simulink model "NEWVSG"  (R2024b)
settings: Solver=FixedStepAuto  StartTime=0.0  StopTime=2  FixedStep=1e-6  RelTol=1e-3
InitFcn:
  | fn=50;
  | Un=24;
  | Sb=100;
  | Qref=1;
  | w0=2*pi*fn;
  | Pref=100;
  | J=0.0002;%典型值0.00002
  | D=0.4;%典型值0.4
  | kp=0.5;%典型值1
  | kv=0.24;%典型值1 对无功调节响应变快，振荡增加
  | kq=0.01;%典型值0.01 增大此值对无功响应没有影响，随意增大会试系统振荡
libraries: spsSeriesRLCBranchLib x6, spsVoltageMeasurementLib x4, slpidlib x2, spsACVoltageSourceLib x1, spsBreakerLib x1, spspowerguiLib x1, spsCurrentMeasurementLib x1, spsDCVoltageSourceLib x1, powerlib_extras x1, simulink x1, spsUniversalBridgeLib x1, spsRMSLib x1
settings Model: Creator=ASUS  LastModifiedBy=ASUS
settings DataIOCC: ReturnWorkspaceOutputs=off

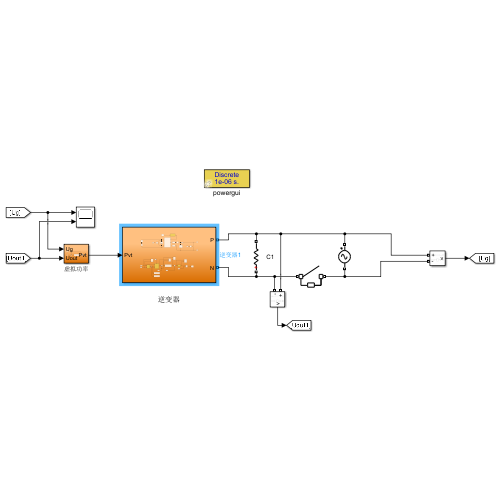
[thumbnail: Simulink's stored preview of the top-level diagram]
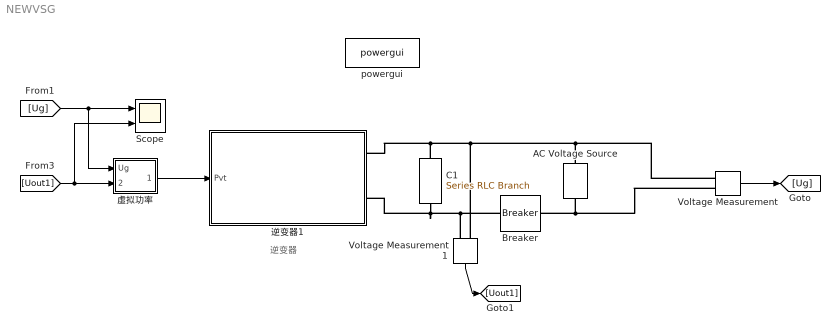
== system NEWVSG ==
  note: 逆变器
  AC Voltage Source : spsACVoltageSourceLib/AC Voltage Source  Amplitude=24*sqrt(2)  Phase=180  Frequency=50  SampleTime=0  Measurements=None  BusType=swing  Pref=10e3  Qref=0  Qmin=-inf  Qmax=+inf
  Breaker : spsBreakerLib/Breaker  InitialState=0  SwitchingTimes=[0.5 1.5 2]  External=off  BreakerResistance=0.01  SnubberResistance=1e6  SnubberCapacitance=inf  Measurements=None  MoreParameters=on  NoBreakLoop=off
  C1 : spsSeriesRLCBranchLib/Series RLC Branch  LConnTagsString=__new0  RConnTagsString=__new0  BranchType=R  Resistance=5  Inductance=0  SetiL0=off  InitialCurrent=0  Capacitance=3e-6  Setx0=off  InitialVoltage=350  Measurements=None
  Scope : Scope  NumInputPorts=2
  Voltage Measurement : spsVoltageMeasurementLib/Voltage Measurement  PhasorSimulation=off  OutputType=Complex  PSBequivalent=0
  Voltage Measurement1 : spsVoltageMeasurementLib/Voltage Measurement  PhasorSimulation=off  OutputType=Complex  PSBequivalent=0
  powergui : spspowerguiLib/powergui  SimulationMode=Discrete  SampleTime=1e-6  frequency=60  Iterations=50  frequencyindice=50  Pbase=100e6  ErrMax=1e-4  UnitsV=kV  UnitsW=MW  buscounter=0  FunctionMessages=off  echomessages=off  EnableUseOfTLC=off  CurrentSourceSwitches=off  DisableSnubberDevices=off  DisableRonSwitches=off  DisableVfSwitches=off  DisplayEquations=off  AutomaticDiscreteSolvers=off  SolverType=Tustin/Backward Euler (TBE)  Interpol=off  ExternalGateDelay=off  methode=off  Ts=0  x0status=blocks  SPID=off  SwTol=0  HookPort=off  NonlinearTolerance=1e-4  nMaxIteration=100  ContinueOnMaxIteration=off  RestoreLinks=warning  ResistiveCurrentMeasurement=off  Frange=[0:2:500]  Ylog=off  Xlog=on  ShowGrid=off  save=off  variable=ZData  structure=QQQQQ  ZoomFFT=off  StartTime=0.5  cycles=15  DisplayStyle=1  fundamental=50  FreqAxis=off  MaxFrequency=1000  frequencyindicesteady=1  RmsSteady=1  display=off
  虚拟功率 : Subsystem
  逆变器1 : Subsystem
      settings: PortSchema="{\"entries\":[{\"content\":{\"sides\":[{\"content\":{},\"type\":\"ConnectorPlacement.EquallySpacedRectSide\",\"uuid\":\"a93680c0-663f-4f34-b987-d4dbc78c4730\"},{\"content\":{\"side\":\"RIGHT\"},\"type\":\"ConnectorPlacement.EquallySpacedRectSide\",\"uuid\":\"c51b779d-273d-4c0b-b109-877d58986348\"},{\"content\":{\"connectorIds\":[\"In1\"],\"side\":\"TOP\"},\"type\":\"ConnectorPlacement.EquallySpacedRectSide\",\"uuid\":\"2562aadc-3010-41da-9435-a9c5d6d596bf\"},{\"content\":{\"connectorIds\":[\"RConn1\",\"RConn2\"],\"side\":\"BOTTOM\"},\"type\":\"ConnectorPlacement.EquallySpacedRectSide\",\"uuid\":\"37d810f6-ab81-4958-8785-8b1d526c8ea4\"}]},\"type\":\"ConnectorPlacement.EquallySpacedConnector\",\"uuid\":\"534c4e7c-1935-4667-a56d-b399c5878ac6\"}],\"packageUris\":[\"http://schema.mathworks.com/mf0/Connector/R2020b\"],\"version\":\"1.0\"}"
  wires:
  虚拟功率/1(Pvt) -> 逆变器1/1(Pvt)
  [Uout1] -> 虚拟功率/2(Uout), Scope/2
  [Ug] -> 虚拟功率/1(Ug), Scope/1
  Voltage Measurement1/1 -> [Uout1]
  Voltage Measurement/1 -> [Ug]
  connections:
  AC Voltage Source/LConn1 -- Breaker/RConn1 -- Voltage Measurement/LConn2
  AC Voltage Source/RConn1 -- 逆变器1/RConn2 -- C1/RConn1 -- Voltage Measurement1/LConn1 -- Voltage Measurement/LConn1
  Breaker/LConn1 -- 逆变器1/RConn1 -- C1/LConn1 -- Voltage Measurement1/LConn2

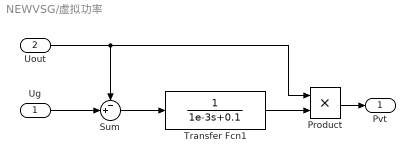
== system NEWVSG/虚拟功率 ==
  Ug : Inport
  Uout : Inport  Port=2
  Product : Product
  Sum : Sum  Inputs=-+|
  Transfer Fcn1 : TransferFcn  Denominator=[1e-3 0.1]
  Pvt : Outport
  wires:
  Transfer Fcn1/1 -> Product/2
  Uout/1 -> Sum/1, Product/1
  Ug/1 -> Sum/2
  Sum/1 -> Transfer Fcn1/1
  Product/1 -> Pvt/1

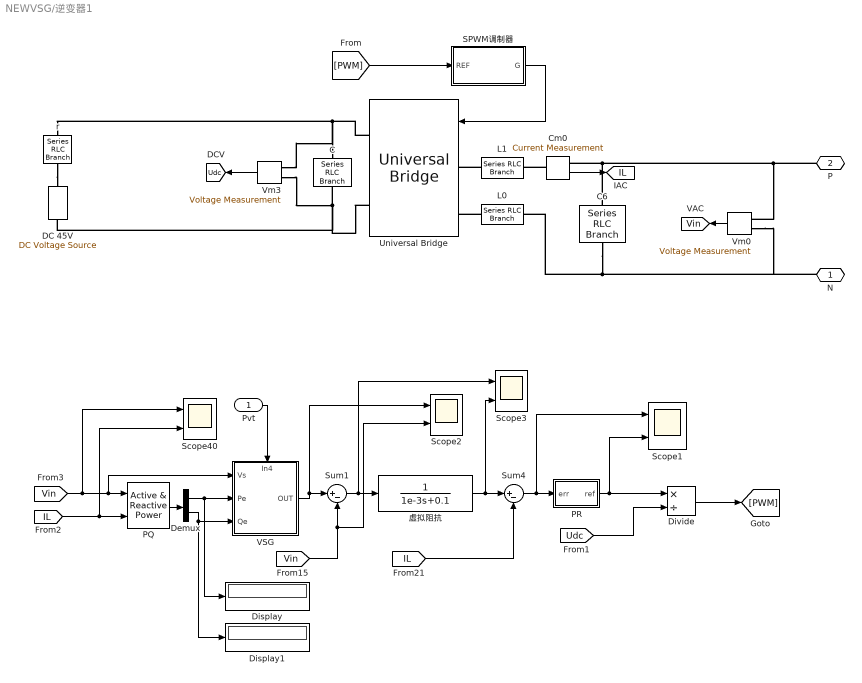
== system NEWVSG/逆变器1 ==
  Pvt : Inport
  C : spsSeriesRLCBranchLib/Series RLC Branch  LConnTagsString=__new0  RConnTagsString=__new0  BranchType=C  Resistance=0.05  Inductance=0  SetiL0=off  InitialCurrent=0  Capacitance=4e-3  Setx0=on  InitialVoltage=45  Measurements=None
  C6 : spsSeriesRLCBranchLib/Series RLC Branch  LConnTagsString=__new0  RConnTagsString=__new0  BranchType=RC  Resistance=1  Inductance=0  SetiL0=off  InitialCurrent=0  Capacitance=3e-6  Setx0=off  InitialVoltage=350  Measurements=None
  Cm0 : spsCurrentMeasurementLib/Current Measurement  PhasorSimulation=off  OutputType=Complex  PSBequivalent=0
  DC 45V : spsDCVoltageSourceLib/DC Voltage Source  Amplitude=45  Measurements=None
  Demux : Demux  Outputs=2
  Display : Display
  Display1 : Display
  Divide : Product  Inputs=*/
  L0 : spsSeriesRLCBranchLib/Series RLC Branch  LConnTagsString=__new0  RConnTagsString=__new0  BranchType=RL  Resistance=81e-3  Inductance=5e-4  SetiL0=off  InitialCurrent=0  Capacitance=inf  Setx0=off  InitialVoltage=0  Measurements=None
  L1 : spsSeriesRLCBranchLib/Series RLC Branch  LConnTagsString=__new0  RConnTagsString=__new0  BranchType=RL  Resistance=81e-3  Inductance=5e-4  SetiL0=off  InitialCurrent=0  Capacitance=inf  Setx0=off  InitialVoltage=0  Measurements=None
  PQ : powerlib_extras/Measurements/Active & Reactive Power  f1=50
  PR : Subsystem  TreatAsAtomicUnit=on  mask{Kp=4, Kr=100, Wc=20, Upper=10000, Lower=-10000}
  SPWM调制器 : Subsystem
  Scope{1..3,40} (4 alike) : Scope  NumInputPorts=2
  Sum1 : Sum  Inputs=|+-
  Sum4 : Sum  Inputs=|+-
  Universal Bridge : spsUniversalBridgeLib/Universal Bridge  Arms=2  SnubberResistance=1e5  SnubberCapacitance=inf  Device=MOSFET / Diodes  Ron=0.01  Lon=0  ForwardVoltages="[  0  0  ]"  ForwardVoltage=0  GTOparameters=[ 10e-6 , 20e-6 ]  IGBTparameters=[ 1e-6 , 2e-6 ]  Measurements=None  Measurements_2=None  converterType=Rectifier
  VSG : Subsystem
      settings: PortSchema="{\"entries\":[{\"content\":{\"sides\":[{\"content\":{\"connectorIds\":[\"In1\",\"In2\",\"In3\"]},\"type\":\"ConnectorPlacement.EquallySpacedRectSide\",\"uuid\":\"aa52da4d-f934-47f0-800a-70195eace23d\"},{\"content\":{\"connectorIds\":[\"Out1\"],\"side\":\"RIGHT\"},\"type\":\"ConnectorPlacement.EquallySpacedRectSide\",\"uuid\":\"90c9e631-faf7-42fe-9625-64aab78a5d50\"},{\"content\":{\"connectorIds\":[\"In4\"],\"side\":\"TOP\"},\"type\":\"ConnectorPlacement.EquallySpacedRectSide\",\"uuid\":\"027d9aee-22b5-4ed3-abeb-2e992649b09d\"}]},\"type\":\"ConnectorPlacement.EquallySpacedConnector\",\"uuid\":\"8c25c37b-9c43-4192-89c9-033fe8e08717\"}],\"packageUris\":[\"http://schema.mathworks.com/mf0/Connector/R2020b\"],\"version\":\"1.0\"}"
  Vm0 : spsVoltageMeasurementLib/Voltage Measurement  PhasorSimulation=off  OutputType=Complex  PSBequivalent=0
  Vm3 : spsVoltageMeasurementLib/Voltage Measurement  PhasorSimulation=off  OutputType=Complex  PSBequivalent=0
  r : spsSeriesRLCBranchLib/Series RLC Branch  LConnTagsString=__new0  RConnTagsString=__new0  BranchType=R  Resistance=0.05  Inductance=0  SetiL0=off  InitialCurrent=0  Capacitance=2e-3  Setx0=on  InitialVoltage=390  Measurements=None
  虚拟阻抗 : TransferFcn  Denominator=[1e-3 0.1]
  N : PMIOPort  Side=Right
  P : PMIOPort  Port=2  Side=Right
  tag scope: IL=global, Udc=global, Vin=global
  wires:
  Vm0/1 -> [Vin]
  Cm0/1 -> [IL]
  Vm3/1 -> [Udc]
  Sum4/1 -> PR/1(err), Scope1/1
  PR/1(ref) -> Divide/1, Scope1/2
  [Udc] -> Divide/2
  [IL] -> Sum4/2
  SPWM调制器/1(G) -> Universal Bridge/1
  [IL] -> PQ/2, Scope40/2
  PQ/1 -> Demux/1
  Sum1/1 -> Scope3/1, 虚拟阻抗/1
  [Vin] -> PQ/1, VSG/1(Vs), Scope40/1
  Demux/1 -> VSG/2(Pe), Display/1
  Demux/2 -> VSG/3(Qe), Display1/1
  [Vin] -> Sum1/2, Scope2/2
  Divide/1 -> [PWM]
  [PWM] -> SPWM调制器/1(REF)
  VSG/1(OUT) -> Scope2/1, Sum1/1
  Pvt/1 -> VSG/4(In4)
  虚拟阻抗/1 -> Scope3/2, Sum4/1
  connections:
  L0/LConn1 -- Universal Bridge/LConn2
  L1/LConn1 -- Universal Bridge/LConn1
  P/RConn1 -- Vm0/LConn1 -- Cm0/RConn1 -- C6/LConn1
  Cm0/LConn1 -- L1/RConn1
  C6/RConn1 -- Vm0/LConn2 -- N/RConn1 -- L0/RConn1
  r/RConn1 -- DC 45V/RConn1
  Vm3/LConn2 -- Universal Bridge/RConn2 -- DC 45V/LConn1 -- C/RConn1
  Universal Bridge/RConn1 -- Vm3/LConn1 -- C/LConn1 -- r/LConn1

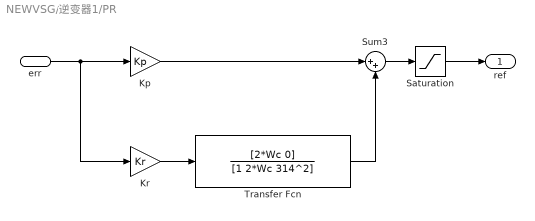
== system NEWVSG/逆变器1/PR ==
  err : Inport
  Kp : Gain  Gain=Kp
  Kr : Gain  Gain=Kr
  Saturation : Saturate  UpperLimit=Upper  LowerLimit=Lower
  Sum3 : Sum  Inputs=|++
  Transfer Fcn : TransferFcn  Numerator=[2*Wc 0]  Denominator=[1 2*Wc 314^2]
  ref : Outport
  wires:
  Kp/1 -> Sum3/1
  Sum3/1 -> Saturation/1
  err/1 -> Kr/1, Kp/1
  Kr/1 -> Transfer Fcn/1
  Transfer Fcn/1 -> Sum3/2
  Saturation/1 -> ref/1

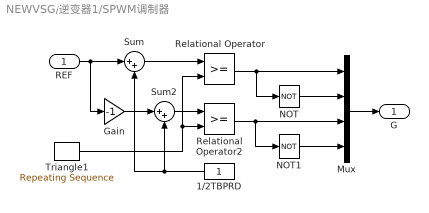
== system NEWVSG/逆变器1/SPWM调制器 ==
  REF : Inport
  1/2TBPRD : Constant
  Gain : Gain  Gain=-1
  Mux : Mux
  NOT : Logic  Operator=NOT  IconShape=distinctive  AllPortsSameDT=off  OutDataTypeStr=boolean
  NOT1 : Logic  Operator=NOT  IconShape=distinctive  AllPortsSameDT=off  OutDataTypeStr=boolean
  Relational Operator : RelationalOperator  OutDataTypeStr=boolean  InputSameDT=off
  Relational Operator2 : RelationalOperator  OutDataTypeStr=boolean  InputSameDT=off
  Sum : Sum  Inputs=|++
  Sum2 : Sum  Inputs=|++
  Triangle1 : simulink/Sources/Repeating Sequence  rep_seq_t=[0 1/16000/2 1/16000]  rep_seq_y=[0 2 0]
  G : Outport
  wires:
  Triangle1/1 -> Relational Operator2/2, Relational Operator/2
  Sum/1 -> Relational Operator/1
  REF/1 -> Gain/1, Sum/1
  Gain/1 -> Sum2/1
  Sum2/1 -> Relational Operator2/1
  1/2TBPRD/1 -> Sum/2, Sum2/2
  Relational Operator/1 -> NOT/1, Mux/1
  NOT/1 -> Mux/2
  Mux/1 -> G/1
  NOT1/1 -> Mux/4
  Relational Operator2/1 -> NOT1/1, Mux/3

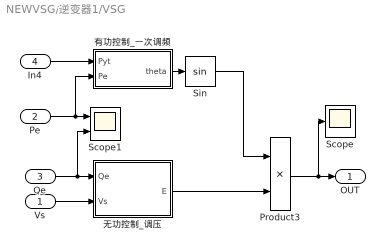
== system NEWVSG/逆变器1/VSG ==
  Vs : Inport
  Pe : Inport  Port=2
  Qe : Inport  Port=3
  In4 : Inport  Port=4
  Product3 : Product
  Scope : Scope
  Scope1 : Scope  NumInputPorts=2
  Sin : Trigonometry
  无功控制_调压 : Subsystem
  有功控制_一次调频 : Subsystem
  OUT : Outport
  wires:
  Pe/1 -> 有功控制_一次调频/2(Pe), Scope1/1
  Product3/1 -> Scope/1, OUT/1
  无功控制_调压/1(E) -> Product3/2
  有功控制_一次调频/1(theta) -> Sin/1
  Sin/1 -> Product3/1
  Qe/1 -> Scope1/2, 无功控制_调压/1(Qe)
  Vs/1 -> 无功控制_调压/2(Vs)
  In4/1 -> 有功控制_一次调频/1(Pyt)

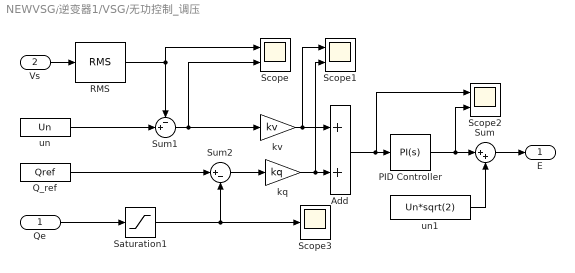
== system NEWVSG/逆变器1/VSG/无功控制_调压 ==
  Qe : Inport
  Vs : Inport  Port=2
  Add : Sum
  PID Controller : slpidlib/PID Controller  Controller=PI  Form=Parallel  TimeDomain=Continuous-time  UseExternalTs=off  SampleTime=-1  IntegratorMethod=Forward Euler  FilterMethod=Forward Euler  ControllerParametersSource=internal  P=0.1  I=50  UseKiTs=off  D=0  UseExternalDerivativeSource=off  N=100  UseFilter=on  TunerSelectOption=Transfer Function Based (PID Tuner App)  InitialConditionSource=internal  InitialConditionForIntegrator=0  InitialConditionForFilter=0  DifferentiatorICPrevScaledInput=0  ExternalReset=none  TrackingMode=off  Kt=1  LimitOutput=off  SatLimitsSource=internal  UpperSaturationLimit=inf  LowerSaturationLimit=-inf  LinearizeAsGain=on  AntiWindupMode=none  Kb=1  LimitIntegrator=off  UpperIntegratorSaturationLimit=inf  LowerIntegratorSaturationLimit=-inf  POutMin=[]  POutMax=[]  IOutMin=[]  IOutMax=[]  DOutMin=[]  DOutMax=[]  NOutMin=[]  NOutMax=[]  SumOutMin=[]  SumOutMax=[]  SaturationOutMin=[]  SaturationOutMax=[]  PParamMin=[]  PParamMax=[]  IParamMin=[]  IParamMax=[]  DParamMin=[]  DParamMax=[]  NParamMin=[]  NParamMax=[]  KbParamMin=[]  KbParamMax=[]  KtParamMin=[]  KtParamMax=[]  KbOutMin=[]  KbOutMax=[]  KtOutMin=[]  KtOutMax=[]  IntegratorOutMin=[]  IntegratorOutMax=[]  FilterOutMin=[]  FilterOutMax=[]  SumI1OutMin=[]  SumI1OutMax=[]  SumI2OutMin=[]  SumI2OutMax=[]  SumI3OutMin=[]  SumI3OutMax=[]  SumI4OutMin=[]  SumI4OutMax=[]  SumDOutMin=[]  SumDOutMax=[]  DifferentiatorOutMin=[]  DifferentiatorOutMax=[]  FilterDiffOutCoefMin=[]  FilterDiffOutCoefMax=[]  ReciprocalOutMin=[]  ReciprocalOutMax=[]  SumDenOutMin=[]  SumDenOutMax=[]  SumNumOutMin=[]  SumNumOutMax=[]  DivideOutMin=[]  DivideOutMax=[]  UdiffTsProdOutMin=[]  UdiffTsProdOutMax=[]  NTsProdOutMin=[]  NTsProdOutMax=[]  UintegralTsProdOutMin=[]  UintegralTsProdOutMax=[]  UngainTsProdOutMin=[]  UngainTsProdOutMax=[]  ClampingZeroOutDataTypeStr=Inherit: Inherit via back propagation  ClampingZeroOutMin=[]  ClampingZeroOutMax=[]  FilterDenConstantOutDataTypeStr=Inherit: Inherit via back propagation  FilterDenConstantOutMin=[]  FilterDenConstantOutMax=[]  PCopyOutDataTypeStr=Inherit: Inherit via back propagation  PCopyOutMin=[]  PCopyOutMax=[]  NCopyOutDataTypeStr=Inherit: Inherit via back propagation  NCopyOutMin=[]  NCopyOutMax=[]  IntegratorContinuousStateAttributes=''  IntegratorStateMustResolveToSignalObject=off  IntegratorRTWStateStorageClass=Auto  FilterContinuousStateAttributes=''  FilterStateMustResolveToSignalObject=off  FilterRTWStateStorageClass=Auto  ParallelPVariant=InternalParameters  IdealPVariant=Disabled  IVariant=InternalParameters  DVariant=Disabled  IntegratorVariant=Continuous  SatVariant=Disabled  AWVariant=Passthrough  PCopyVariant=Disabled  TRVariant=Disabled  FdbkBlocksVariant=Forward  IdealPFdbkVariant=Disabled  SatFdbkVariant=Disabled  DerivativeFilterVariant=Disabled  NVariant=Disabled  NCopyVariant=Disabled_SignalSpec  FilterICVariant=Disabled  IntegratorICVariant=InternalICs  ExternalResetVariant=Disabled  TRSumVariant=Passthrough  SumFdbkVariant=Disabled  SumVariant=Sum_PI  TsampFilterVariant=InternalTs  TsampNgainVariant=Passthrough  TsampIntegralVariant=Disabled_SignalSpec  ExternalSaturationOutDataTypeStr=Inherit: Same as second input  DerivativeSourceVariant=Disabled  PreIntVariant=InternalPreInt
  Q_ref : Constant  Value=Qref
  RMS : spsRMSLib/RMS  TrueRMS=on  Freq=50  RMSInit=24  Ts=0
  Saturation1 : Saturate  UpperLimit=100  LowerLimit=-100
  Scope : Scope  NumInputPorts=2
  Scope1 : Scope  NumInputPorts=2
  Scope2 : Scope  NumInputPorts=2
  Scope3 : Scope
  Sum : Sum  Inputs=|++
  Sum1 : Sum  Inputs=-+|
  Sum2 : Sum  Inputs=|+-
  kq : Gain  Gain=kq
  kv : Gain  Gain=kv
  un : Constant  Value=Un
  un1 : Constant  Value=Un*sqrt(2)
  E : Outport
  wires:
  Vs/1 -> RMS/1
  Sum/1 -> E/1
  kv/1 -> Scope1/1, Add/1
  un1/1 -> Sum/2
  Add/1 -> Scope2/1, PID Controller/1
  un/1 -> Sum1/2
  RMS/1 -> Scope/1, Sum1/1
  kq/1 -> Scope1/2, Add/2
  PID Controller/1 -> Scope2/2, Sum/1
  Sum2/1 -> kq/1
  Sum1/1 -> Scope/2, kv/1
  Q_ref/1 -> Sum2/1
  Qe/1 -> Saturation1/1
  Saturation1/1 -> Sum2/2, Scope3/1

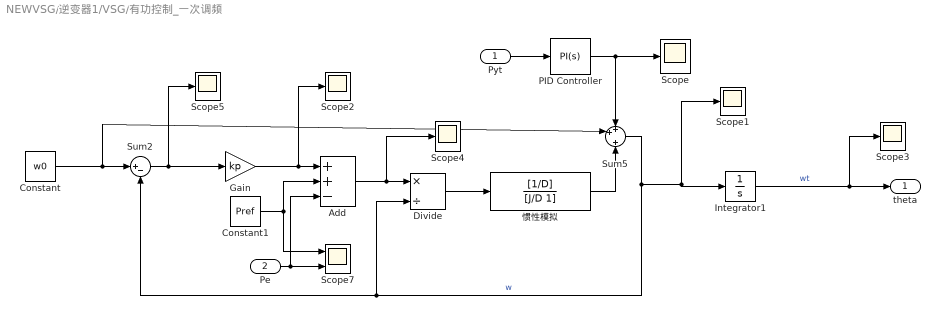
== system NEWVSG/逆变器1/VSG/有功控制_一次调频 ==
  Pyt : Inport
  Pe : Inport  Port=2
  Add : Sum  Inputs=++-
  Constant : Constant  Value=w0
  Constant1 : Constant  Value=Pref
  Divide : Product  Inputs=*/
  Gain : Gain  Gain=kp
  Integrator1 : Integrator  WrapState=on  WrappedStateUpperValue=2*pi  WrappedStateLowerValue=0
  PID Controller : slpidlib/PID Controller  Controller=PI  Form=Parallel  TimeDomain=Continuous-time  UseExternalTs=off  SampleTime=-1  IntegratorMethod=Forward Euler  FilterMethod=Forward Euler  ControllerParametersSource=internal  P=0.04  I=0  UseKiTs=off  D=0  UseExternalDerivativeSource=off  N=100  UseFilter=on  TunerSelectOption=Transfer Function Based (PID Tuner App)  InitialConditionSource=internal  InitialConditionForIntegrator=0  InitialConditionForFilter=0  DifferentiatorICPrevScaledInput=0  ExternalReset=none  TrackingMode=off  Kt=1  LimitOutput=on  SatLimitsSource=internal  UpperSaturationLimit=30  LowerSaturationLimit=-30  LinearizeAsGain=on  AntiWindupMode=none  Kb=1  LimitIntegrator=off  UpperIntegratorSaturationLimit=inf  LowerIntegratorSaturationLimit=-inf  POutMin=[]  POutMax=[]  IOutMin=[]  IOutMax=[]  DOutMin=[]  DOutMax=[]  NOutMin=[]  NOutMax=[]  SumOutMin=[]  SumOutMax=[]  SaturationOutMin=[]  SaturationOutMax=[]  PParamMin=[]  PParamMax=[]  IParamMin=[]  IParamMax=[]  DParamMin=[]  DParamMax=[]  NParamMin=[]  NParamMax=[]  KbParamMin=[]  KbParamMax=[]  KtParamMin=[]  KtParamMax=[]  KbOutMin=[]  KbOutMax=[]  KtOutMin=[]  KtOutMax=[]  IntegratorOutMin=[]  IntegratorOutMax=[]  FilterOutMin=[]  FilterOutMax=[]  SumI1OutMin=[]  SumI1OutMax=[]  SumI2OutMin=[]  SumI2OutMax=[]  SumI3OutMin=[]  SumI3OutMax=[]  SumI4OutMin=[]  SumI4OutMax=[]  SumDOutMin=[]  SumDOutMax=[]  DifferentiatorOutMin=[]  DifferentiatorOutMax=[]  FilterDiffOutCoefMin=[]  FilterDiffOutCoefMax=[]  ReciprocalOutMin=[]  ReciprocalOutMax=[]  SumDenOutMin=[]  SumDenOutMax=[]  SumNumOutMin=[]  SumNumOutMax=[]  DivideOutMin=[]  DivideOutMax=[]  UdiffTsProdOutMin=[]  UdiffTsProdOutMax=[]  NTsProdOutMin=[]  NTsProdOutMax=[]  UintegralTsProdOutMin=[]  UintegralTsProdOutMax=[]  UngainTsProdOutMin=[]  UngainTsProdOutMax=[]  ClampingZeroOutDataTypeStr=Inherit: Inherit via back propagation  ClampingZeroOutMin=[]  ClampingZeroOutMax=[]  FilterDenConstantOutDataTypeStr=Inherit: Inherit via back propagation  FilterDenConstantOutMin=[]  FilterDenConstantOutMax=[]  PCopyOutDataTypeStr=Inherit: Inherit via back propagation  PCopyOutMin=[]  PCopyOutMax=[]  NCopyOutDataTypeStr=Inherit: Inherit via back propagation  NCopyOutMin=[]  NCopyOutMax=[]  IntegratorContinuousStateAttributes=''  IntegratorStateMustResolveToSignalObject=off  IntegratorRTWStateStorageClass=Auto  FilterContinuousStateAttributes=''  FilterStateMustResolveToSignalObject=off  FilterRTWStateStorageClass=Auto  ParallelPVariant=InternalParameters  IdealPVariant=Disabled  IVariant=InternalParameters  DVariant=Disabled  IntegratorVariant=Continuous  SatVariant=Enabled  AWVariant=Passthrough  PCopyVariant=Disabled  TRVariant=Disabled  FdbkBlocksVariant=Forward  IdealPFdbkVariant=Disabled  SatFdbkVariant=Disabled  DerivativeFilterVariant=Disabled  NVariant=Disabled  NCopyVariant=Disabled_SignalSpec  FilterICVariant=Disabled  IntegratorICVariant=InternalICs  ExternalResetVariant=Disabled  TRSumVariant=Passthrough  SumFdbkVariant=Disabled  SumVariant=Sum_PI  TsampFilterVariant=InternalTs  TsampNgainVariant=Passthrough  TsampIntegralVariant=Disabled_SignalSpec  ExternalSaturationOutDataTypeStr=Inherit: Same as second input  DerivativeSourceVariant=Disabled  PreIntVariant=InternalPreInt
  Scope{,1..5} (6 alike) : Scope
  Scope7 : Scope  NumInputPorts=2
  Sum2 : Sum  Inputs=|+-
  Sum5 : Sum  Inputs=++|+
  惯性模拟 : TransferFcn  Numerator=[1/D]  Denominator=[J/D 1]
  theta : Outport
  wires:
  Integrator1/1 -> theta/1, Scope3/1  "wt"
  Sum5/1 -> Scope1/1, Integrator1/1, Divide/2, Sum2/2  "w"
  Constant/1 -> Sum5/2, Sum2/1
  Sum2/1 -> Gain/1, Scope5/1
  Gain/1 -> Add/1, Scope2/1
  Constant1/1 -> Scope7/1, Add/2
  Pe/1 -> Scope7/2, Add/3
  Add/1 -> Scope4/1, Divide/1
  Pyt/1 -> PID Controller/1
  PID Controller/1 -> Sum5/1, Scope/1
  Divide/1 -> 惯性模拟/1
  惯性模拟/1 -> Sum5/3
